simulink model "SOC_callibration"  (R2021a)
settings: Solver=VariableStepAuto  StartTime=0.0  StopTime=60*30*5  RelTol=1e-3
values from neighbouring files (symbols this model uses):
  initialCurrent = 40*5    (= 200)    [SOC_callibration_script.m]
  initialSOC = 80    [SOC_callibration_script.m]
  period = 60*60    (= 3600)    [SOC_callibration_script.m]
  T = 1    [SOC_callibration_script.m]
undefined symbols (not defined in the file or in its folder): Ion, Lithium
libraries: spsBatteryLib x1, spsControlledCurrentSourceLib x1, simulink x1, spspowerguiLib x1
settings Model: Creator=peter  LastModifiedBy=peter

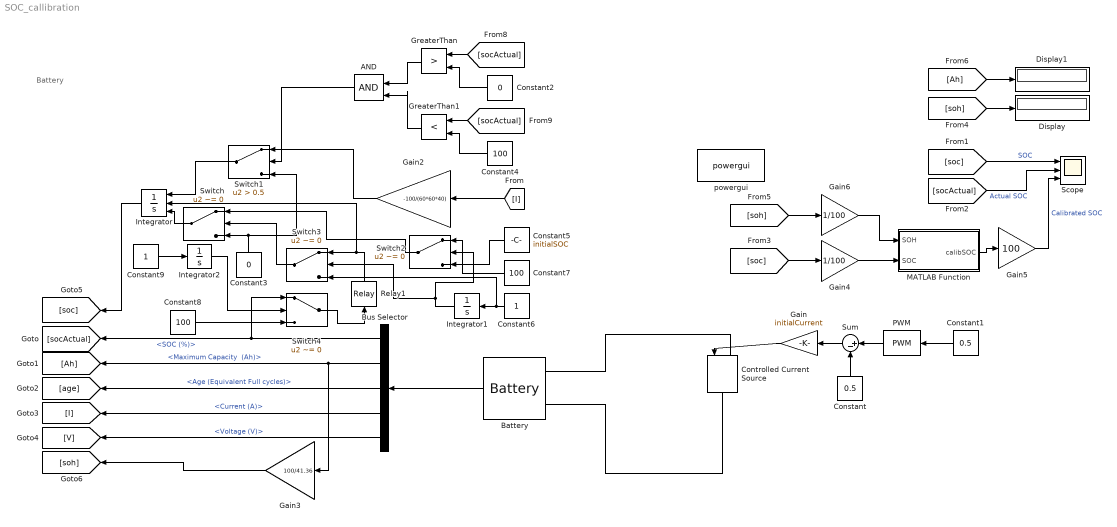
== system SOC_callibration ==
  note: Battery
  AND : Logic  IconShape=distinctive  AllPortsSameDT=off  OutDataTypeStr=boolean
  Battery : spsBatteryLib/Battery  BatType=Lithium-Ion  ShowTempParam=off  ThermalPreset=no  ShowAgeParam=on  NomV=72  NomQ=40  SOC=initialSOC  Batt_Tr=30  PresetModel=on  MaxQ=40  MinV=54  FullV=83.8071  Dis_rate=17.3913  R=0.018  Normal_OP=36.1739  expZone="[77.7878      1.96522]"  current=[6.5 13 32.5]  Units=Ampere-hour  Tci=20  NomT=20  T2=-30  MaxQ2=4.8  FullV2=7.1  Normal_OP2=5.655  expZone2="[6.58           1]"  Rca=0.6  ti=2000  Dp=0  Neq0=300  Tsim=1e6  Ta1=25  Qeol=5.4*0.9  Reol=0.013333*1.2  Char_age=[2.3478, 3]  Dis_age=[2.3478, 10]  N1=1500  N2=10500  N3=1000  N4=1400  Ta2=45  N5=950
  Bus Selector : BusSelector  OutputSignals="SOC (%),Maximum Capacity  (Ah),Age (Equivalent Full cycles),Current (A),Voltage (V)"
  Constant : Constant  Value=0.5  SampleTime=T
  Constant1 : Constant  Value=0.5  SampleTime=T
  Constant2 : Constant  Value=0  SampleTime=T
  Constant3 : Constant  Value=0  SampleTime=T
  Constant4 : Constant  Value=100  SampleTime=T
  Constant5 : Constant  Value=initialSOC  SampleTime=T
  Constant6 : Constant  SampleTime=T
  Constant7 : Constant  Value=100  SampleTime=T
  Constant8 : Constant  Value=100  SampleTime=T
  Constant9 : Constant  SampleTime=T
  Controlled Current Source : spsControlledCurrentSourceLib/Controlled Current Source  Initialize=on  Source_Type=AC  Amplitude=0  Phase=0  Frequency=0  Measurements=None
  Display : Display
  Display1 : Display
  Gain : Gain  Gain=initialCurrent
  Gain2 : Gain  Gain=-100/(60*60*40)
  Gain3 : Gain  Gain=100/41.36
  Gain4 : Gain  Gain=1/100
  Gain5 : Gain  Gain=100
  Gain6 : Gain  Gain=1/100
  GreaterThan : RelationalOperator  Operator=>  OutDataTypeStr=boolean  RndMeth=Simplest
  GreaterThan1 : RelationalOperator  Operator=<  OutDataTypeStr=boolean  RndMeth=Simplest
  Integrator : Integrator  ExternalReset=either  InitialConditionSource=external  InitialCondition=100  UpperSaturationLimit=36.49*60*60  LowerSaturationLimit=0
  Integrator1 : Integrator
  Integrator2 : Integrator
  MATLAB Function : MATLAB Function  TreatAsAtomicUnit=on
  PWM : simulink/Discontinuities/PWM  DisableCoverage=on  Period=period  DisallowZeroDutyCycle=off  RunAtFixedTimeIntervals=off  SampleTime=0.1
  Relay1 : Relay  OnSwitchValue=99.9999  OffSwitchValue=0.0001
  Scope : Scope  NumInputPorts=3
  Sum : Sum  Inputs=|+-
  Switch : Switch  Criteria=u2 ~= 0  Threshold=0.5
  Switch1 : Switch  Criteria=u2 > Threshold  Threshold=0.5
  Switch2 : Switch  Criteria=u2 ~= 0
  Switch3 : Switch  Criteria=u2 ~= 0
  Switch4 : Switch  Criteria=u2 ~= 0
  powergui : spspowerguiLib/powergui  Priority=1  SimulationMode=Discrete  SampleTime=T  frequency=60  Iterations=50  frequencyindice=0  Pbase=100e6  ErrMax=1e-4  UnitsV=kV  UnitsW=MW  buscounter=0  FunctionMessages=off  echomessages=off  EnableUseOfTLC=off  CurrentSourceSwitches=off  DisableSnubberDevices=off  DisableRonSwitches=off  DisableVfSwitches=off  DisplayEquations=off  AutomaticDiscreteSolvers=off  SolverType=Tustin/Backward Euler (TBE)  Interpol=off  ExternalGateDelay=off  methode=off  Ts=100  x0status=blocks  SPID=on  SwTol=0  HookPort=off  NonlinearTolerance=1e-4  nMaxIteration=100  ContinueOnMaxIteration=off  RestoreLinks=warning  ResistiveCurrentMeasurement=off  Frange=[0:2:500]  Ylog=off  Xlog=on  ShowGrid=off  save=off  variable=ZData  structure=0  ZoomFFT=off  StartTime=0.0  cycles=1  DisplayStyle=1  fundamental=60  FreqAxis=off  MaxFrequency=1000  frequencyindicesteady=1  RmsSteady=1  display=off
  wires:
  Battery/1 -> Bus Selector/1
  Bus Selector/1 -> [socActual], Switch4/1  "<SOC (%)>"
  Bus Selector/3 -> [age]  "<Age (Equivalent Full cycles)>"
  Gain/1 -> Controlled Current Source/1
  PWM/1 -> Sum/1
  Constant/1 -> Sum/2
  Constant1/1 -> PWM/1
  Sum/1 -> Gain/1
  Bus Selector/2 -> [Ah], Gain3/1  "<Maximum Capacity  (Ah)>"
  Bus Selector/4 -> [I]  "<Current (A)>"
  Bus Selector/5 -> [V]  "<Voltage (V)>"
  Gain3/1 -> [soh]
  [soc] -> Scope/1  "SOC"
  [socActual] -> Scope/2  "Actual SOC"
  [soc] -> Gain4/1
  Gain5/1 -> Scope/3  "Calibrated SOC"
  Gain4/1 -> MATLAB Function/2(SOC)
  MATLAB Function/1(calibSOC) -> Gain5/1
  [soh] -> Display/1
  [soh] -> Gain6/1
  Gain6/1 -> MATLAB Function/1(SOH)
  [Ah] -> Display1/1
  Integrator/1 -> [soc]
  [I] -> Gain2/1
  Relay1/1 -> Integrator/2, Switch3/1
  Switch/1 -> Integrator/3
  Constant5/1 -> Switch2/3
  Constant3/1 -> Switch1/3, Switch/3
  Gain2/1 -> Switch1/1
  Switch1/1 -> Integrator/1
  [socActual] -> GreaterThan/1
  Constant2/1 -> GreaterThan/2
  Constant4/1 -> GreaterThan1/2
  [socActual] -> GreaterThan1/1
  GreaterThan/1 -> AND/1
  GreaterThan1/1 -> AND/2
  Constant6/1 -> Switch3/3, Integrator1/1
  Switch2/1 -> Switch/1
  Constant7/1 -> Switch2/1
  Integrator1/1 -> Switch3/2, Switch2/2
  Switch3/1 -> Switch/2
  AND/1 -> Switch1/2
  Constant8/1 -> Switch4/3
  Integrator2/1 -> Switch4/2
  Constant9/1 -> Integrator2/1
  Switch4/1 -> Relay1/1
  connections:
  Battery/LConn1 -- Controlled Current Source/LConn1
  Controlled Current Source/RConn1 -- Battery/LConn2

== matlab function SOC_callibration/MATLAB Function ==
  settings: updateMethod=DISCRETE
  data: SOH input; SOC input; calibSOC output
function calibSOC = fcn(SOH, SOC)
persistent bChange

SOC_MARGIN = 0.01;
bSOH = SOH;

if isempty(bChange)
   bChange = 0;
end

% change detect
if SOC<=(0.0+SOC_MARGIN)
    bChange = +1;% rising from 0% SOC
elseif SOC>=(1.0-SOC_MARGIN)
    bChange = -1;% falling from 100% SOC
end

% SOC Calibration
% For falling from 100% SOC    : newSOC = (SOC-(1-SOH))/SOH
% For rising from 0% SOC       : newSOC = SOC/SOH

bNewSOC = SOC;
if bChange~=0 %Update only if we actually know the rising from 0% or falling from 100%
    if bChange == -1
       bNewSOC = (SOC-(1-bSOH))/bSOH; 
    elseif bChange == 1
        bNewSOC = SOC/bSOH; 
    end
end

calibSOC = bNewSOC;
